simulink model "encode_decode_withoutAlarms_correction1"  (R2022a)
settings: Solver=VariableStepAuto  StartTime=0.0  StopTime=200  RelTol=1e-3
libraries: simulink x7, spsSampleandHoldLib x3
settings Model: Creator=mluser  LastModifiedBy=mluser
settings ModelReferenceCC: EnableRefExpFcnMdlSchedulingChecks=off
settings RTWCC: Description=Generic Real-Time Target

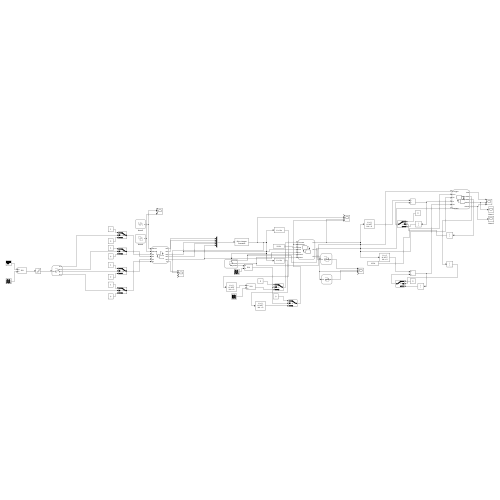
[thumbnail: Simulink's stored preview of the top-level diagram]
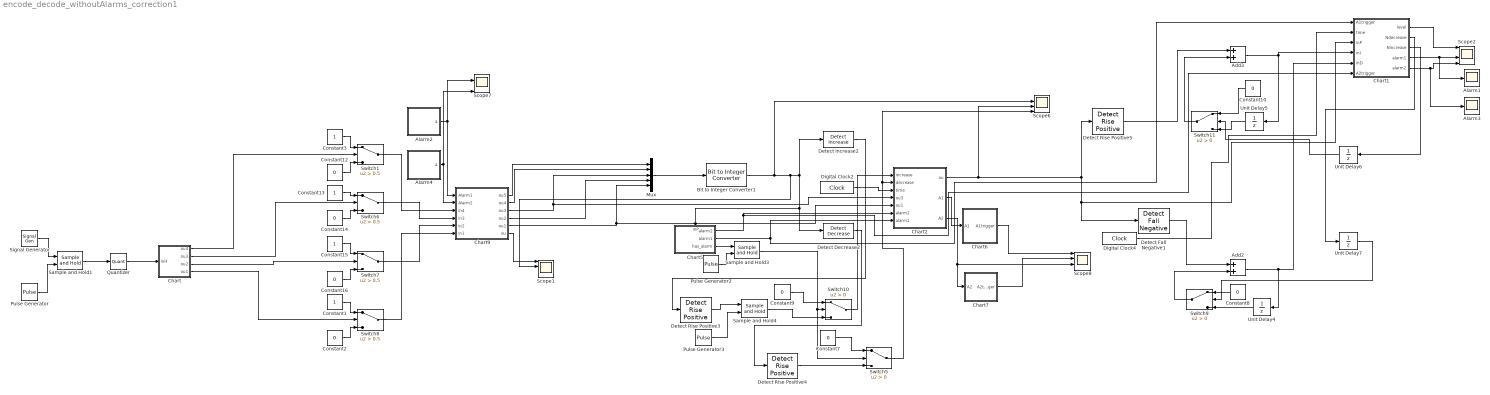
== system encode_decode_withoutAlarms_correction1 ==
  Add2 : Sum
  Add3 : Sum
  Alarm1 : Scope
  Alarm2 : Stateflow chart  TreatAsAtomicUnit=on
  Alarm3 : Scope
  Alarm4 : Stateflow chart  TreatAsAtomicUnit=on
  Bit to Integer Converter1 : simulink/Logic and Bit Operations/Bit to Integer Converter  nbits=5  bitOrder=MSB first  signedOutputValues=Unsigned  outDtype=Inherit via internal rule  outDtypeSigned=Inherit via internal rule
  Chart : Stateflow chart  TreatAsAtomicUnit=on
      settings: PortSchema="{\"entries\":[{\"content\":{\"sides\":[{\"content\":{\"connectorIds\":[\"In1\"]},\"type\":\"ConnectorPlacement.EquallySpacedRectSide\",\"uuid\":\"aaeedc4a-65ef-4d8f-ba01-1ddc4e011816\"},{\"content\":{\"connectorIds\":[\"Out2\",\"Out1\",\"Out3\",\"Out4\"],\"side\":\"RIGHT\"},\"type\":\"ConnectorPlacement.EquallySpacedRectSide\",\"uuid\":\"bfc75945-f598-4b29-99c0-df6bb3f156b5\"},{\"content\":{\"connectorIds\":[],\"side\":\"TOP\"},\"type\":\"ConnectorPlacement.EquallySpacedRectSide\",\"uuid\":\"e78d9c07-753c-4a5b-aa63-095c584c660c\"}]},\"type\":\"ConnectorPlacement.EquallySpacedConnector\",\"uuid\":\"f46ef6be-e67f-4bb7-838b-d108f8d3e6f5\"}],\"packageUris\":[\"http://schema.mathworks.com/mf0/Connector/R2020b\"],\"version\":\"1.0\"}"
  Chart1 : Stateflow chart  TreatAsAtomicUnit=on
  Chart2 : Stateflow chart  TreatAsAtomicUnit=on
  Chart5 : Stateflow chart  TreatAsAtomicUnit=on
      settings: PortSchema="{\"entries\":[{\"content\":{\"sides\":[{\"content\":{\"connectorIds\":[]},\"type\":\"ConnectorPlacement.EquallySpacedRectSide\",\"uuid\":\"5c3dd9c4-40fc-475e-8fc4-53a3db762fc4\"},{\"content\":{\"connectorIds\":[\"Out1\",\"Out2\",\"Out3\"],\"side\":\"RIGHT\"},\"type\":\"ConnectorPlacement.EquallySpacedRectSide\",\"uuid\":\"288f4f63-e8ff-4ace-a90f-863d45689e1d\"},{\"content\":{\"connectorIds\":[\"In1\"],\"side\":\"TOP\"},\"type\":\"ConnectorPlacement.EquallySpacedRectSide\",\"uuid\":\"c4c1c7c7-df9c-4060-9033-81f7d31c6bbf\"}]},\"type\":\"ConnectorPlacement.EquallySpacedConnector\",\"uuid\":\"fd27b28a-c6e9-46f2-af96-6d8beda93238\"}],\"packageUris\":[\"http://schema.mathworks.com/mf0/Connector/R2020b\"],\"version\":\"1.0\"}"
  Chart6 : Stateflow chart  TreatAsAtomicUnit=on
  Chart7 : Stateflow chart  TreatAsAtomicUnit=on
  Chart9 : Stateflow chart  TreatAsAtomicUnit=on
      settings: PortSchema="{\"entries\":[{\"content\":{\"sides\":[{\"content\":{\"connectorIds\":[\"In2\",\"In1\",\"In4\",\"In6\",\"In5\",\"In3\"]},\"type\":\"ConnectorPlacement.EquallySpacedRectSide\",\"uuid\":\"927bfff6-0efb-434d-9b76-b310eeccee4d\"},{\"content\":{\"connectorIds\":[\"Out4\",\"Out3\",\"Out2\",\"Out1\",\"Out5\",\"Out6\"],\"side\":\"RIGHT\"},\"type\":\"ConnectorPlacement.EquallySpacedRectSide\",\"uuid\":\"ec167fcb-832d-4548-a5f6-e3acff823e9a\"},{\"content\":{\"connectorIds\":[],\"side\":\"TOP\"},\"type\":\"ConnectorPlacement.EquallySpacedRectSide\",\"uuid\":\"7cc63ad6-e1ff-415f-bbd0-59110a67e519\"}]},\"type\":\"ConnectorPlacement.EquallySpacedConnector\",\"uuid\":\"a8329d4d-4148-47f0-9db5-a03c892023c4\"}],\"packageUris\":[\"http://schema.mathworks.com/mf0/Connector/R2020b\"],\"version\":\"1.0\"}"
  Constant{1,3,13,15} (4 alike) : Constant
  Constant{2,7..10,12,14,16} (8 alike) : Constant  Value=0
  Detect Decrease2 : simulink/Logic and Bit Operations/Detect Decrease  vinit=0.0  OutDataTypeStr=boolean
  Detect Increase2 : simulink/Logic and Bit Operations/Detect Increase  vinit=0.0  OutDataTypeStr=boolean
  Detect Fall Negative1 : simulink/Logic and Bit Operations/Detect Fall Negative  vinit=0  OutDataTypeStr=boolean
  Detect Rise Positive3 : simulink/Logic and Bit Operations/Detect Rise Positive  vinit=0  OutDataTypeStr=boolean
  Detect Rise Positive4 : simulink/Logic and Bit Operations/Detect Rise Positive  vinit=0  OutDataTypeStr=boolean
  Detect Rise Positive5 : simulink/Logic and Bit Operations/Detect Rise Positive  vinit=0  OutDataTypeStr=boolean
  Digital Clock2 : DigitalClock  SampleTime=0.01
  Digital Clock4 : DigitalClock  SampleTime=0.01
  Mux : Mux  Inputs=5
  Pulse Generator : DiscretePulseGenerator  PulseType=Time based  Period=0.01  PulseWidth=5  PhaseDelay=0.1
  Pulse Generator2 : DiscretePulseGenerator  PulseType=Time based  Period=0.2  PulseWidth=5  PhaseDelay=0.1
  Pulse Generator3 : DiscretePulseGenerator  PulseType=Time based  Period=0.05  PulseWidth=5  PhaseDelay=0.1
  Quantizer : Quantizer
  Sample and Hold1 : spsSampleandHoldLib/Sample and Hold  ic=0  Ts=0.1
  Sample and Hold3 : spsSampleandHoldLib/Sample and Hold  ic=0  Ts=0.1
  Sample and Hold4 : spsSampleandHoldLib/Sample and Hold  ic=0  Ts=0.1
  Scope{1..2,6..8} (5 alike) : Scope  NumInputPorts=4
  Signal Generator : SignalGenerator  Amplitude=40  Frequency=0.02  Units=rad/sec
  Switch{1,6..8} (4 alike) : Switch  Criteria=u2 > Threshold  Threshold=0.5  SaturateOnIntegerOverflow=off  InputSameDT=off
  Switch{5,9..11} (4 alike) : Switch  Criteria=u2 > Threshold  SaturateOnIntegerOverflow=off  InputSameDT=off
  Unit Delay{4..7} (4 alike) : UnitDelay  SampleTime=-1  HasFrameUpgradeWarning=on
  wires:
  Chart6/1(A1trigger) -> Scope8/1
  Constant10/1 -> Switch11/1
  Sample and Hold3/1 -> Switch5/2, Switch10/2
  Chart5/2(alarm1) -> Chart1/1(A1trigger), Chart2/7(alarm1)
  Digital Clock4/1 -> Chart1/2(time)
  Unit Delay4/1 -> Switch9/3
  Constant8/1 -> Switch9/1
  Detect Rise Positive3/1 -> Sample and Hold4/1
  Add2/1 -> Chart1/5(inD), Unit Delay4/1
  Switch11/1 -> Add3/2
  Switch5/1 -> Scope6/4, Chart2/2(decrease)
  Sample and Hold4/1 -> Switch10/3
  Detect Increase2/1 -> Detect Rise Positive3/1
  Mux/1 -> Bit to Integer Converter1/1
  Detect Fall Negative1/1 -> Add2/1
  Pulse Generator2/1 -> Sample and Hold3/2
  Chart7/1(A2trigger) -> Scope8/2
  Chart2/3(A2) -> Scope8/3, Chart7/1(A2)
  Chart2/1(ou) -> Scope6/3, Chart1/3(inP), Detect Fall Negative1/1, Detect Rise Positive5/1
  Switch10/1 -> Chart2/1(increase)
  Unit Delay5/1 -> Switch11/3
  Pulse Generator3/1 -> Sample and Hold4/2
  Detect Rise Positive4/1 -> Switch5/3
  Constant9/1 -> Switch10/1
  Detect Rise Positive5/1 -> Add3/1
  Chart2/2(A1) -> Chart6/1(A1)
  Unit Delay6/1 -> Switch11/2
  Bit to Integer Converter1/1 -> Scope6/2, Scope1/2, Chart5/1(inP), Detect Decrease2/1, Detect Increase2/1
  Unit Delay7/1 -> Switch9/2
  Chart5/3(has_alarm) -> Sample and Hold3/1
  Constant7/1 -> Switch5/1
  Switch9/1 -> Add2/2
  Detect Decrease2/1 -> Detect Rise Positive4/1
  Chart5/1(alarm2) -> Chart1/6(A2trigger), Chart2/6(alarm2)
  Digital Clock2/1 -> Chart2/3(time)
  Chart/3(ou2) -> Switch7/2
  Switch6/1 -> Chart9/6(in3)
  Constant3/1 -> Switch1/1
  Sample and Hold1/1 -> Quantizer/1
  Signal Generator/1 -> Sample and Hold1/1
  Quantizer/1 -> Chart/1(inH)
  Switch1/1 -> Chart9/4(in4)
  Chart/2(ou4) -> Switch1/2
  Pulse Generator/1 -> Sample and Hold1/2
  Switch7/1 -> Chart9/5(in2)
  Constant2/1 -> Switch8/3
  Constant16/1 -> Switch7/3
  Constant1/1 -> Switch8/1
  Switch8/1 -> Chart9/3(in1)
  Constant12/1 -> Switch1/3
  Chart/1(ou3) -> Switch6/2
  Constant14/1 -> Switch6/3
  Constant13/1 -> Switch6/1
  Chart/4(ou1) -> Switch8/2
  Constant15/1 -> Switch7/1
  Chart9/4(ou5) -> Mux/1
  Chart9/3(ou4) -> Mux/2
  Chart9/2(ou3) -> Mux/3, Chart2/4(ou3)
  Chart9/1(ou2) -> Mux/4
  Chart9/5(ou1) -> Chart2/5(ou1), Mux/5
  Chart9/6(ou) -> Scope1/1
  Alarm2/1(a) -> Chart9/2(Alarm1), Scope7/2
  Alarm4/1(a) -> Chart9/1(Alarm2), Scope7/4
  Add3/1 -> Unit Delay5/1, Chart1/4(inI)
  Chart1/4(alarm1) -> Alarm1/1, Scope2/3
  Chart1/5(alarm2) -> Alarm3/1, Scope2/4
  Chart1/1(level) -> Scope2/1
  Chart1/3(Nincrease) -> Unit Delay6/1
  Chart1/2(Ndecrease) -> Unit Delay7/1

== stateflow chart encode_decode_withoutAlarms_correction1/Chart1 ==
  state Decoder
    entry:
    state Normal_water_level_measure
      entry:
      state state1
        entry:
        level=0;
        Ndecrease=0;
        Nincrease=0;
      state initial
        entry:
        Ndecrease=0;
        Nincrease=0;
      state state2
        entry:
        level=1;
        Ndecrease=0;
        Nincrease=0;
      state state3
        entry:
        level=2;
        Ndecrease=0;
        Nincrease=0;
      state state5
        entry:
        level=4;
        Ndecrease=0;
        Nincrease=0;
      state state4
        entry:
        level=3;
        Nincrease=0;
        Ndecrease=0;
      (default) -> initial
      state1 -> state2 : [time>=1&&inP==1&&inI<=1]
      initial -> state1 [order 2] : [inP==1]
          | {Ndecrease=0;
          | Nincrease=0;}
      (junction 15) -> state1 : {Ndecrease=1;
          | Nincrease=1;}
      initial -> state5 [order 1] : [time<1&&inP==-1]
      state2 -> (junction 15) [order 2] : [time>=1&&inP==-1&&inD==3]
      state3 -> state2 [order 2] : [time>=1&&inP==-1&&inD==3]
      state2 -> state3 [order 1] : [time>=1&&inP==1&&inI<=2]
      state4 -> state3 [order 2] : [time>=1&&inP==-1&&inD<=3]
      state3 -> state4 [order 1] : [time>=1&&inP==1&&inI==2]
      state4 -> (junction 20) [order 1] : [time>=1&&inP==1&&inI>=3]
      (junction 20) -> state5 : {Ndecrease=1;
          | Nincrease=1;}
      state5 -> state4 : [time>=1&&inP==-1&&inD<=2]
    state Alarm_triggering
      entry:
      state A1
        entry:
        alarm1=1;
      state Alarm_b
        entry: alarm1=0;
        alarm2=0;
      state A2
        entry:
        alarm2=1;
        Ndecrease=0;
        Nincrease=0;
      (default) -> Alarm_b
      Alarm_b -> A1 [order 2] : [A1trigger==1]
      A1 -> Alarm_b : [A1trigger==0]
      A2 -> Alarm_b : [A2trigger==0]
      Alarm_b -> A2 [order 1] : [A2trigger==1]
    (default) -> Normal_water_level_measure
    Normal_water_level_measure -> Alarm_triggering : [A1trigger==1||A2trigger==1]
        | {Ndecrease=0;Nincrease=0;}
    Alarm_triggering -> Normal_water_level_measure : [A1trigger==0&&A2trigger==0]
        | {Nincrease=0;Ndecrease=0;}
  (default) -> Decoder
  data: A1trigger input; time input; inP input; inI input; inD input; A2trigger input; level output; Ndecrease output; Nincrease output; alarm1 output; alarm2 output

== stateflow chart encode_decode_withoutAlarms_correction1/Chart2 ==
  (junction 100) -> (junction 140) [order 2] : [alarm1==1]
  (junction 140) -> (junction 131) : {A1=1;}
  (default) -> (junction 100) : {A1=0;A2=0;}
  (junction 100) -> (junction 95) [order 1]
  (junction 131) -> (junction 128)
  (junction 134) -> (junction 128) : {A2=1;}
  (junction 95) -> (junction 134) [order 2] : [alarm2==1]
  (junction 128) -> (junction 44)
  (junction 95) -> (junction 3) [order 1]
  (junction 3) -> (junction 28) [order 2] : [increase==1&&time>0]
  (junction 28) -> (junction 44) : {ou=1;}
  (junction 3) -> (junction 10) [order 1]
  (junction 44) -> (junction 43)
  (junction 10) -> (junction 8) [order 1] : [decrease==1&&time>0]
  (junction 8) -> (junction 43) : {ou=-1;}
  (junction 10) -> (junction 71) [order 2]
  (junction 43) -> (junction 72)
  (junction 71) -> (junction 73) [order 1] : [time==0&&ou3==1]
  (junction 73) -> (junction 72) : {ou=1;}
  (junction 71) -> (junction 78) [order 2]
  (junction 72) -> (junction 80)
  (junction 78) -> (junction 79) [order 1] : [time==0&&ou1==0]
  (junction 79) -> (junction 80) : {ou=-1;}
  (junction 78) -> (junction 90) [order 2]
  (junction 80) -> (junction 88)
  (junction 89) -> (junction 88) : {ou=0}
  (junction 90) -> (junction 89) : [increase==0&&decrease==0]
  data: increase input; decrease input; ou output; time input; ou3 input; ou1 input; alarm2 input; A1 output; A2 output; alarm1 input

== stateflow chart encode_decode_withoutAlarms_correction1/Chart ==
  (default) -> (junction 3) : {ou1=0;
      | ou2=0;
      | ou3=0;
      | ou4=0;
      | }
  (junction 3) -> (junction 28) [order 2] : [inH==0]
  (junction 28) -> (junction 44) : {ou1=0;ou2=0;ou3=0;ou4=0;}
  (junction 3) -> (junction 10) [order 1]
  (junction 44) -> (junction 43)
  (junction 10) -> (junction 8) [order 1] : [inH<=10]
  (junction 8) -> (junction 43) : {ou1=1;ou2=0;ou3=0;ou4=0;}
  (junction 10) -> (junction 12) [order 2]
  (junction 43) -> (junction 42)
  (junction 16) -> (junction 42) : {ou1=1;ou2=1;ou3=0;ou4=0;}
  (junction 12) -> (junction 16) [order 1] : [inH>10&&inH<=20]
  (junction 42) -> (junction 41)
  (junction 12) -> (junction 19) [order 2]
  (junction 19) -> (junction 18) [order 1] : [inH>20&&inH<=30]
  (junction 18) -> (junction 41) : {ou1=1;ou2=1;ou3=1;ou4=0;}
  (junction 41) -> (junction 63)
  (junction 19) -> (junction 61) [order 2]
  (junction 61) -> (junction 62) : [inH>30]
  (junction 62) -> (junction 63) : {ou1=1;ou2=1;ou3=1;ou4=1;}
  data: ou3 output; ou4 output; ou2 output; ou1 output; inH input

== stateflow chart encode_decode_withoutAlarms_correction1/Alarm2 ==
  state begin
    du:a=0;
  state end
    du:a=1;
  (default) -> begin
  begin -> end : after(100,sec)
  end -> begin : after(0.2,sec)
  data: a output

== stateflow chart encode_decode_withoutAlarms_correction1/Chart5 ==
  state alarm1
    entry:
    alarm1=1;
    has_alarm=1;
    after(0.2,sec);
  state alarm_detect
    entry:
    alarm1=0;
    alarm2=0;
    has_alarm=0;
  state alarm2
    entry:
    alarm2=1;
    has_alarm=1;
    after(0.2,sec);
  alarm_detect -> alarm1 [order 1] : [inP==31]
  (default) -> alarm_detect
  alarm1 -> alarm_detect : [inP<20]
  alarm_detect -> alarm2 [order 2] : [inP==30]
  alarm2 -> alarm_detect : [inP<20]
  data: inP input; alarm2 output; alarm1 output; has_alarm output

== stateflow chart encode_decode_withoutAlarms_correction1/Chart6 ==
  state begin
    entry:
    A1trigger=0;
  state end
    entry:
    A1trigger=1;
    after(0.2,sec);
  (default) -> begin : {A1trigger=0;}
  begin -> end : [A1==1]
  end -> begin : [A1==0]
  data: A1trigger output; A1 input

== stateflow chart encode_decode_withoutAlarms_correction1/Chart7 ==
  state begin
    entry:
    A2trigger=0;
  state end
    entry:
    A2trigger=1;
    after(0.2,sec);
  (default) -> begin : {A2trigger=0;}
  begin -> end : [A2==1]
  end -> begin : [A2==0]
  data: A2trigger output; A2 input

== stateflow chart encode_decode_withoutAlarms_correction1/Chart9 ==
  state Water
    state q1
      entry:ou1=0;ou2=0;
      ou3=0;ou4=0;ou5=0;
    state q2
      entry:ou1=1;ou2=0;
      ou3=0;ou4=0;ou5=0;
    state Input
      entry:
    state q3
      entry:ou1=1;ou2=1;
      ou3=0;ou4=0;ou5=0;
    state q4
      entry:ou1=1;ou2=1;
      ou3=1;ou4=0;ou5=0;
    state q5
      entry:ou1=1;ou2=1;
      ou3=1;ou4=1;ou5=0;
    Input -> q1 [order 1] : [in1==1&&in2==0&&in3==0&&in4==0]
        | {ou=0;}
    q1 -> q2 : [in1==1&&in2==0&&in3==0&&in4==0]
        | {ou=1;}
    q2 -> q1 [order 1] : [in1==0&&in2==0&&in3==0&&in4==0]
        | {ou=0;}
    q2 -> q3 [order 2] : [in1==1&&in2==1&&in3==0&&in4==0]
        | {ou=1;}
    q3 -> q2 [order 1] : [in1==1&&in2==0&&in3==0&&in4==0]
        | {ou=0;}
    (default) -> Input
    Input -> q5 [order 2] : [in1==1&&in2==1&&in3==1&&in4==1]
        | {ou=1;}
    q3 -> q4 [order 2] : [in1==1&&in2==1&&in3==1&&in4==0]
        | {ou=1;}
    q4 -> q3 [order 1] : [in1==1&&in2==1&&in3==0&&in4==0]
        | {ou=0;}
    q4 -> q5 [order 2] : [in1==1&&in2==1&&in3==1&&in4==1]
        | {ou=1;}
    q5 -> q4 : [in1==1&&in2==1&&in3==1&&in4==0]
        | {ou=0;}
  state Alarm
    state A1
      entry:
      ou1=1;
      ou2=1;
      ou3=1;
      ou4=1;ou5=1;
    state Alarm_b
      entry:
    state A2
      entry:
      ou1=1;
      ou2=1;
      ou3=1;
      ou4=1;ou5=1;
    (default) -> Alarm_b
    Alarm_b -> A1 [order 2] : [Alarm1==1]
    A1 -> Alarm_b : [Alarm1==0]
    A2 -> Alarm_b : [Alarm2==0]
    Alarm_b -> A2 [order 1] : [Alarm2==1]
  (default) -> Water
  Water -> Alarm : [Alarm1==1||Alarm2==1]
  Alarm -> Water : [Alarm1==0&&Alarm2==0]
  data: Alarm2 input; Alarm1 input; in1 input; in4 input; in2 input; in3 input; ou2 output; ou3 output; ou4 output; ou5 output; ou1 output; ou output

== stateflow chart encode_decode_withoutAlarms_correction1/Alarm4 ==
  state begin
    du:a=0;
  state end
    du:a=1;
  (default) -> begin
  begin -> end : after(70,sec)
  end -> begin : after(0.2,sec)
  data: a output
